simulink model "Robot_Physics_Model_slx"  (R2025b)
settings: Solver=VariableStepAuto  StartTime=0.0  StopTime=10.0  RelTol=1e-3
values from neighbouring files (symbols this model uses):
  den_plant = [1  0  -Alpha_n]    [Parameters_Script.m]
  num_plant = [K_motor]    [Parameters_Script.m]
libraries: simulink x1
settings Model: Creator=Steven Ayman  LastModifiedBy=Steven Ayman

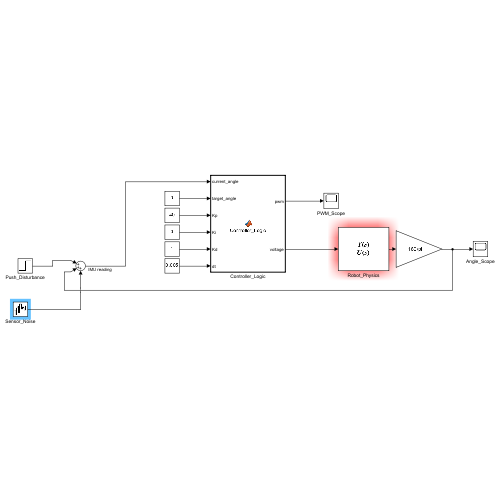
[thumbnail: Simulink's stored preview of the top-level diagram]
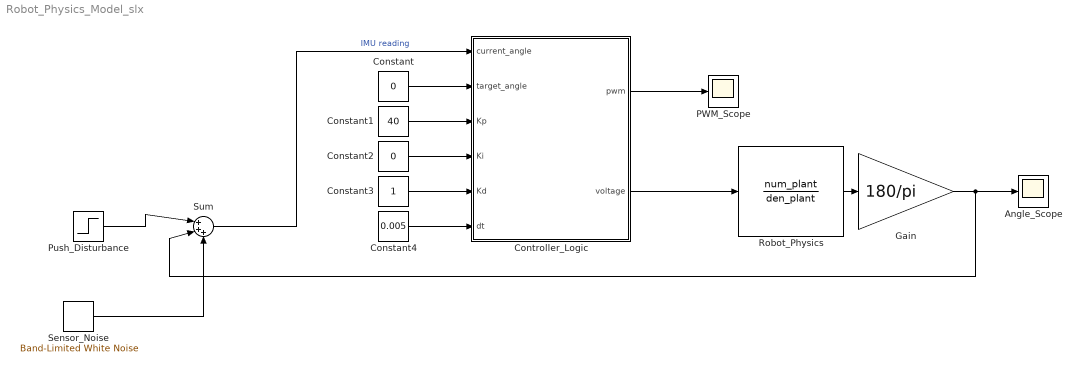
== system Robot_Physics_Model_slx ==
  Angle_Scope : Scope
      settings: ActiveDisplayYMinimum=-0.26744846645837289  ActiveDisplayYMaximum=0.18594676460386156
  Constant : Constant  Value=0
  Constant1 : Constant  Value=40
  Constant2 : Constant  Value=0
  Constant3 : Constant
  Constant4 : Constant  Value=0.005
  Controller_Logic : MATLAB Function  TreatAsAtomicUnit=on  SystemSampleTime=0.005
  Gain : Gain  Gain=180/pi
  PWM_Scope : Scope
      settings: ActiveDisplayYMinimum=-50.782601244972525  ActiveDisplayYMaximum=52.899850161116674
  Push_Disturbance : Step  After=0  SampleTime=0
  Robot_Physics : TransferFcn  Numerator=num_plant  Denominator=den_plant
  Sensor_Noise : simulink/Sources/Band-Limited White Noise  Cov=[0.00001]  Ts=0.1  seed=[23341]
  Sum : Sum  Inputs=|+++
  wires:
  Push_Disturbance/1 -> Sum/1
  Sensor_Noise/1 -> Sum/3
  Sum/1 -> Controller_Logic/1(current_angle)  "IMU reading"
  Constant/1 -> Controller_Logic/2(target_angle)
  Constant4/1 -> Controller_Logic/6(dt)
  Constant3/1 -> Controller_Logic/5(Kd)
  Constant2/1 -> Controller_Logic/4(Ki)
  Constant1/1 -> Controller_Logic/3(Kp)
  Controller_Logic/2(voltage) -> Robot_Physics/1
  Controller_Logic/1(pwm) -> PWM_Scope/1
  Gain/1 -> Sum/2, Angle_Scope/1
  Robot_Physics/1 -> Gain/1

== matlab function Robot_Physics_Model_slx/Controller_Logic ==
  data: current_angle input; pwm output; target_angle input; Kp input; Ki input; Kd input; dt input; voltage output
function [pwm, voltage] = Controller_Logic(current_angle, target_angle, Kp, Ki, Kd, dt)
    % PERSISTENT VARIABLES (Memory like 'static' in C++)
    persistent errorSum lastError
    if isempty(errorSum)
        errorSum = 0;
        lastError = 0;
    end

    % 1. ERROR CALC
    error = target_angle - current_angle;
    
    % 2. INTEGRAL (with anti-windup from your code)
    errorSum = errorSum + error * dt;
    if errorSum > 200, errorSum = 200; end
    if errorSum < -200, errorSum = -200; end
    
    % 3. DERIVATIVE
    dError = (error - lastError) / dt;
    lastError = error;
    
    % 4. PID OUTPUT
    pidOutput = (Kp * error) + (Ki * errorSum) + (Kd * dError);
    
    % 5. AGGRESSIVE BOOST (Your custom logic)
    if error > 8
        pidOutput = pidOutput + 40;
    elseif error < -8
        pidOutput = pidOutput - 40;
    end
    
    % 6. DEADZONE COMPENSATION & LIMITS
    % Constrain to 255
    if pidOutput > 255, pidOutput = 255; end
    if pidOutput < -255, pidOutput = -255; end
    
    % "Anti-Deadzone" (Your code: force 35 if between 0 and 35)
    if (pidOutput > 0 && pidOutput < 35)
        pwm = 35;
    elseif (pidOutput < 0 && pidOutput > -35)
        pwm = -35;
    else
        pwm = pidOutput;
    end
    
    % Convert PWM (0-255) to approximate Voltage (0-12V) for physics model
    voltage = (pwm / 255) * 12; 
end
